simulink model "ex4_8b"  (R2020b)
settings: Solver=VariableStepAuto  StartTime=0.0  StopTime=10.0  RelTol=1e-3
libraries: dsparch4 x1
settings Model: Creator=seojoon  LastModifiedBy=seojoon

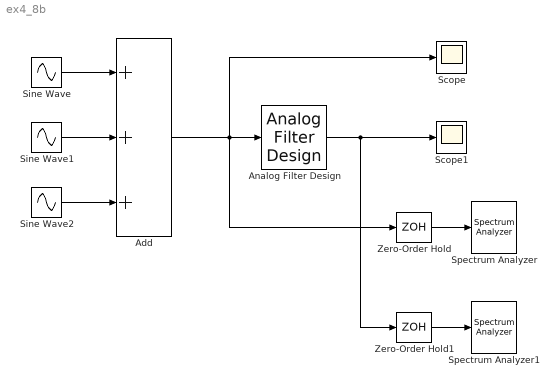
== system ex4_8b ==
  Add : Sum  Inputs=+++
  Analog Filter Design : dsparch4/Analog Filter Design  method=Butterworth  filttype=Lowpass  N=8  Wlo=2*pi*110  Whi=80  Rp=2  Rs=40
  Scope : Scope
  Scope1 : Scope
  Sine Wave : Sin  Amplitude=10  Frequency=2*pi*50  SampleTime=0
  Sine Wave1 : Sin  Amplitude=10  Frequency=2*pi*100  Phase=pi/2  SampleTime=0
  Sine Wave2 : Sin  Amplitude=-10  Frequency=2*pi*200  SampleTime=0
  Spectrum Analyzer : SpectrumAnalyzer
  Spectrum Analyzer1 : SpectrumAnalyzer
  Zero-Order Hold : ZeroOrderHold  SampleTime=1e-3
  Zero-Order Hold1 : ZeroOrderHold  SampleTime=1e-3
  wires:
  Sine Wave2/1 -> Add/3
  Add/1 -> Scope/1, Analog Filter Design/1, Zero-Order Hold/1
  Zero-Order Hold/1 -> Spectrum Analyzer/1
  Sine Wave1/1 -> Add/2
  Sine Wave/1 -> Add/1
  Zero-Order Hold1/1 -> Spectrum Analyzer1/1
  Analog Filter Design/1 -> Zero-Order Hold1/1, Scope1/1
